simulink model "Utkarsh_2005574_W1_P4_Ref_Model"  (R2020b)
settings: Solver=FixedStepDiscrete  StartTime=0.0  StopTime=10.0  FixedStep=0.2  RelTol=1e-3
settings Model: Creator=home  LastModifiedBy=home
settings DataIOCC: SaveOutput=off  SaveTime=off

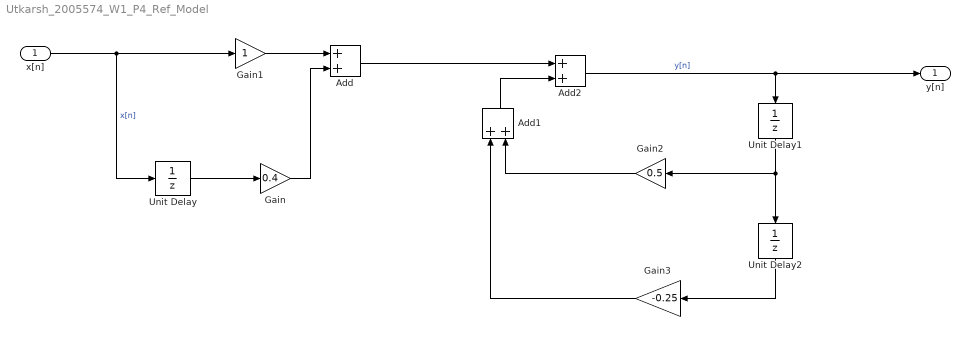
== system Utkarsh_2005574_W1_P4_Ref_Model ==
  x[n] : Inport  OutDataTypeStr=double  PortDimensions=1  SampleTime=[0.20000000000000001,0]
  Add : Sum
  Add1 : Sum
  Add2 : Sum
  Gain : Gain  Gain=0.4
  Gain1 : Gain
  Gain2 : Gain  Gain=0.5
  Gain3 : Gain  Gain=-0.25
  Unit Delay : UnitDelay  SampleTime=-1  HasFrameUpgradeWarning=on
  Unit Delay1 : UnitDelay  SampleTime=-1  HasFrameUpgradeWarning=on
  Unit Delay2 : UnitDelay  SampleTime=-1  HasFrameUpgradeWarning=on
  y[n] : Outport  OutDataTypeStr=double  PortDimensions=1  SampleTime=[0.20000000000000001,0]
  wires:
  Add/1 -> Add2/1
  Unit Delay1/1 -> Gain2/1, Unit Delay2/1
  Gain1/1 -> Add/1
  Unit Delay2/1 -> Gain3/1
  x[n]/1 -> Gain1/1, Unit Delay/1  "x[n]"
  Gain2/1 -> Add1/2
  Add1/1 -> Add2/2
  Gain/1 -> Add/2
  Unit Delay/1 -> Gain/1
  Add2/1 -> Unit Delay1/1, y[n]/1  "y[n]"
  Gain3/1 -> Add1/1
